simulink model "Lagrange"  (R2025b)
settings: Solver=ode45  StartTime=0.0  StopTime=80  RelTol=1e-3  EnableMultiTasking=on
values from neighbouring files (symbols this model uses):
  parameters = [m1,m2,I1,I2,a1,a2,l1,l2,g]    [Lag_main.m]
  q_final = [[pi/2;0],[0;0],[0;0]]    [Lag_main.m]
  q_mid_1 = [[-pi/2;3*pi/4],[0;0],[0;0]]    [Lag_main.m]
  q_mid_2 = [[pi/4;3*pi/4],[0;0],[0;0]]    [Lag_main.m]
  q_start = [[0;0],[0;0],[0;0]]    [Lag_main.m]
  statei = [[0;0],[0;0],[0;0]]    [Lag_main.m]
settings Model: Creator=RIKEN
settings SolverCC: AlgebraicLoopSolver=TrustRegion
settings DataIOCC: LimitDataPoints=on  SaveFormat=Array  ReturnWorkspaceOutputs=off
settings OptimizationCC: ExpressionDepthLimit=2147483647.0  LifeSpan=inf
settings DebuggingCC: UnderspecifiedInitializationDetection=Classic  MergeDetectMultiDrivingBlocksExec=none  UnconnectedInputMsg=warning  UnconnectedOutputMsg=warning  UnconnectedLineMsg=warning  StateNameClashWarn=warning  SFUnexpectedBacktrackingDiag=warning  SFNoUnconditionalDefaultTransitionDiag=warning  SFExecutionAtInitializationDiag=none  ArithmeticOperatorsInVariantConditions=warning
settings HardwareCC: ProdBitPerPointer=32.0  ProdBitPerSizeT=32.0  ProdBitPerPtrDiffT=32.0  ProdLargestAtomicFloat=None  ProdIntDivRoundTo=Undefined  ProdEndianess=Unspecified  ProdWordSize=32.0  ProdHWDeviceType=32-bit Generic
settings ModelReferenceCC: EnableRefExpFcnMdlSchedulingChecks=on  PropagateSignalLabelsOutOfModel=off
settings SFSimCC: SimUseLocalCustomCode=off  CustomCodeUndefinedFunction=UseInterfaceOnly
settings RTWCC: RTWUseLocalCustomCode=off  GPUComputeCapability=3.5
settings CodeAppCC: StateflowObjectComments=on
settings GRTTargetCC: TargetLangStandard=C89/C90 (ANSI)
settings ConfigComp: CovMetricSettings=dw  CovSaveCumulativeToWorkspaceVar=on  CovSaveSingleToWorkspaceVar=on  CovExternalEMLEnable=off

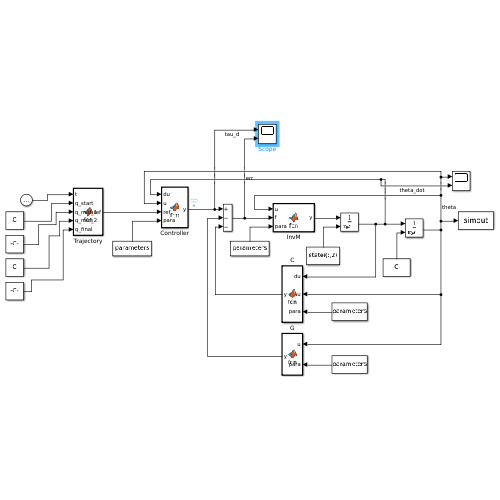
[thumbnail: Simulink's stored preview of the top-level diagram]
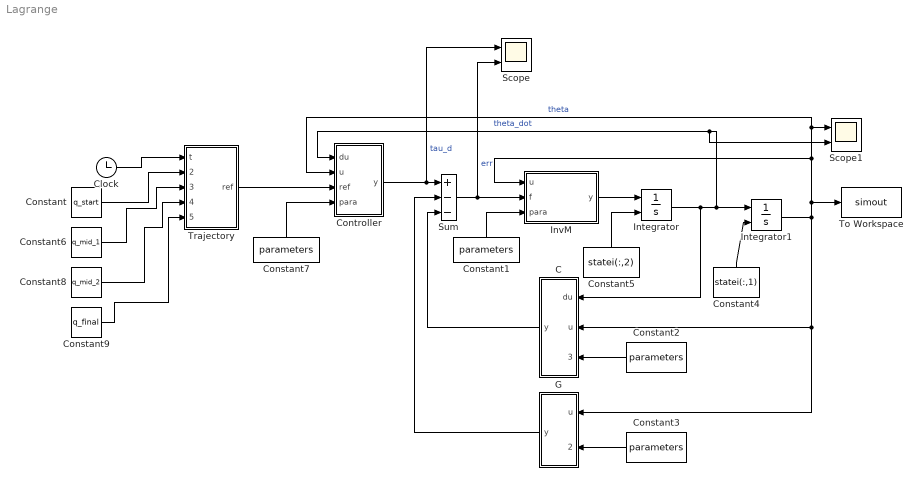
== system Lagrange ==
  C : MATLAB Function  TreatAsAtomicUnit=on
  Clock : Clock
  Constant : Constant  Value=q_start
  Constant{1..3,7} (4 alike) : Constant  Value=parameters
  Constant4 : Constant  Value=statei(:,1)
  Constant5 : Constant  Value=statei(:,2)
  Constant6 : Constant  Value=q_mid_1
  Constant8 : Constant  Value=q_mid_2
  Constant9 : Constant  Value=q_final
  Controller : MATLAB Function  TreatAsAtomicUnit=on
  G : MATLAB Function  TreatAsAtomicUnit=on
  Integrator : Integrator  InitialConditionSource=external
  Integrator1 : Integrator  InitialConditionSource=external
  InvM : MATLAB Function  TreatAsAtomicUnit=on
  Scope : Scope  NumInputPorts=2
      settings: ActiveDisplayYMinimum=-0.039978084493380368  ActiveDisplayYMaximum=0.0529456061820336
  Scope1 : Scope  NumInputPorts=2
      settings: ActiveDisplayYMinimum=-2.3224118929092938  ActiveDisplayYMaximum=6.9240990802161173
  Sum : Sum  Inputs=+--
  To Workspace : ToWorkspace  VariableName=simout  SaveFormat=Timeseries  SampleTime=-1
  Trajectory : MATLAB Function  TreatAsAtomicUnit=on
  wires:
  Controller/1(y) -> Scope/1, Sum/1  "tau_d"
  Sum/1 -> Scope/2, InvM/2(f)  "err"
  InvM/1(y) -> Integrator/1
  G/1(y) -> Sum/2
  C/1(y) -> Sum/3
  Constant1/1 -> InvM/3(para)
  Constant2/1 -> C/3(para)
  Constant3/1 -> G/2(para)
  Constant4/1 -> Integrator1/2
  Constant5/1 -> Integrator/2
  Constant7/1 -> Controller/4(para)
  Integrator1/1 -> To Workspace/1, Controller/2(u), Scope1/1, InvM/1(u), G/1(u), C/2(u)  "theta"
  Integrator/1 -> Scope1/2, Controller/1(du), Integrator1/1, C/1(du)  "theta_dot"
  Clock/1 -> Trajectory/1(t)
  Trajectory/1(ref) -> Controller/3(ref)
  Constant/1 -> Trajectory/2(q_start)
  Constant6/1 -> Trajectory/3(q_mid_1)
  Constant8/1 -> Trajectory/4(q_mid_2)
  Constant9/1 -> Trajectory/5(q_final)

== matlab function Lagrange/C ==
  data: du input; y output; u input; para input
function y = fcn(du,u,para)
%入力：各関節の回転速度
%      各関節の回転角度
%      システムに関するパラメータ
%出力：遠心力・コリオリ力
% C(theta,dtheta)
m2=para(2);
a1=para(5);
l2=para(8);
y1=-m2*a1*l2*sin(u(2))*(2*du(1)*du(2)+du(2)^2);
y2=m2*a1*l2*sin(u(2))*du(1)^2;
y = [y1;y2];

== matlab function Lagrange/InvM ==
  data: u input; f input; y output; para input
function y = fcn(u,f,para)
%入力：各関節の回転角度
%     トルク
%     システムに関するパラメータ
%出力：各関節の回転加速度
%Inverse M(theta)
m1=para(1);
m2=para(2);
I1=para(3);
I2=para(4);
a1=para(5);
l1=para(7);
l2=para(8);
g=para(9);
M11=I1+I2+m1*l1^2+m2*(a1^2+2*a1*l2*cos(u(2))+l2^2);
M12=I2+m2*(a1*l2*cos(u(2))+l2^2);
M21=M12;
M22=I2+m2*l2^2;
y = [M11,M12;M21,M22]\f;

== matlab function Lagrange/G ==
  data: u input; y output; para input
function y = fcn(u,para)
%入力：各関節の回転角度
%      システムに関するパラメータ
%出力：重力
% G(theta)
m1=para(1);
m2=para(2);
a1=para(5);
l1=para(7);
l2=para(8);
g=para(9);
y1=m1*g*l1*cos(u(1))+m2*g*(a1*cos(u(1))+l2*cos(u(1)+u(2)));
y2=m2*g*l2*cos(u(1)+u(2));
y = [y1;y2];

== matlab function Lagrange/Trajectory ==
  settings: updateMethod=CONTINUOUS
  data: t input; q_start input; ref output size=[2, 3] [..3]; q_mid_1 input; q_mid_2 input; q_final input
function ref = fcn(t, q_start,q_mid_1,q_mid_2,q_final)
ref = zeros(2,3);
tmp = zeros(3,2);
coef = zeros(3,2);
poly = zeros(3,3);
% ---------------- Segment timings ----------------
alpha = 1;
T1 = 10*alpha;           % duration of segment 1
T2 = 20*alpha;           % end time of segment 2
T3 = 40*alpha;           % end time of segment 3 (total)

%Ts = T3;
%tau = t;
%q_goal = q_final;
if t < T1
    q_goal = q_mid_1;
    tau     = t;
    Ts      = T1;
elseif t < T2
    q_start = q_mid_1;
    q_goal  = q_mid_2;
    tau     = t - T1;
    Ts      = T2 - T1;
elseif t < T3
    q_start = q_mid_2;
    q_goal  = q_final;
    tau     = t - T2;
    Ts      = T3 - T2;
else
    q_start = q_final;
    q_goal  = q_final;
    tau     = t;
    Ts      = 1; 
end

% ---------- Quintic coefficients per segment ----------
A = [Ts^5    Ts^4    Ts^3;
     5*Ts^4  4*Ts^3  3*Ts^2;
     20*Ts^3 12*Ts^2 6*Ts];

coef = A \ (q_goal' - q_start');   

poly = [tau^5 tau^4 tau^3;
        5*tau^4 4*tau^3 3*tau^2;
        20*tau^3 12*tau^2 6*tau];  

tmp = poly * coef;                 
tmp = tmp + q_start';
ref = tmp.';   

end

== matlab function Lagrange/Controller ==
  data: du input; u input; y output; ref input; para input
function y = fcn(du,u,ref,para)
%入力：各関節の回転速度
%      各関節の回転角度
%      各関節の参照回転角度
%      システムに関するパラメータ
%出力：トルク
m1=para(1);
m2=para(2);
I1=para(3);
I2=para(4);
a1=para(5);
l1=para(7);
l2=para(8);
g=para(9);

%D=100*eye(2);  %微分制御のゲイン
%K=100*eye(2);  %比例制御のゲイン

D=10*eye(2);  %微分制御のゲイン
K=10*eye(2);  %比例制御のゲイン

%慣性力の係数
M11=I1+I2+m1*l1^2+m2*(a1^2+2*a1*l2*cos(u(2))+l2^2);
M12=I2+m2*(a1*l2*cos(u(2))+l2^2);
M21=M12;
M22=I2+m2*l2^2;
qref2dot=ref(:,3); %参照回転加速度
qrefdot=ref(:,2);  %参照回転速度
qref=ref(:,1);     %参照回転角度

%遠心力・コリオリ力
C1=-m2*a1*l2*sin(u(2))*(2*du(1)*du(2)+du(2)^2);
C2=m2*a1*l2*sin(u(2))*du(1)^2;
%重力
G1=m1*g*l1*cos(u(1))+m2*g*(a1*cos(u(1))+l2*cos(u(1)+u(2)));
G2=m2*g*l2*cos(u(1)+u(2));
%y = [C1;C2]+[G1;G2]+...
%    [M11,M12;M21,M22]*(qref2dot+D*(qrefdot-du)+K*(qref-u));
y = [M11,M12;M21,M22]*(qref2dot+D*(qrefdot-du)+K*(qref-u));
